simulink model "DockingSimulationModel"  (R2024b)
settings: Solver=VariableStepAuto  StartTime=0.0  StopTime=10.0  RelTol=1e-3

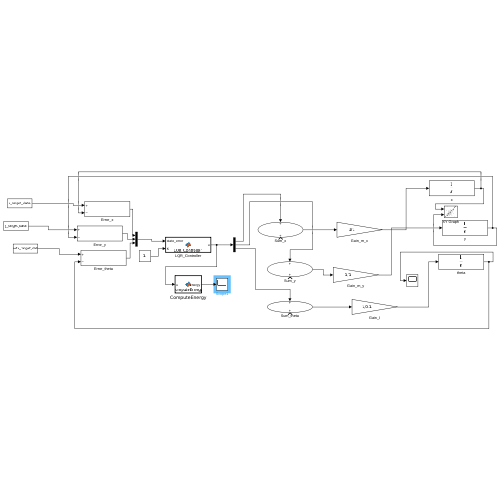
[thumbnail: Simulink's stored preview of the top-level diagram]
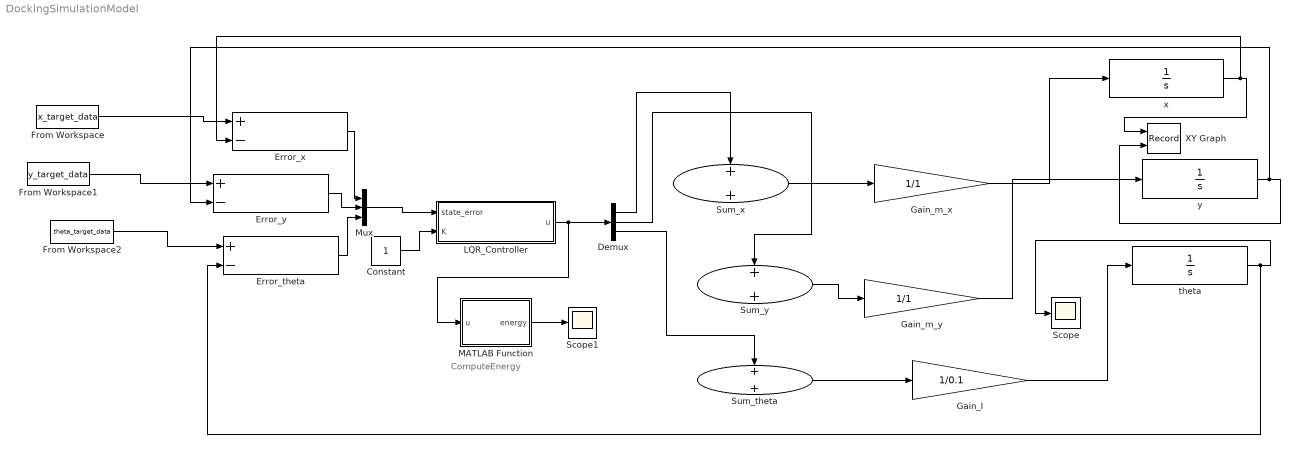
== system DockingSimulationModel ==
  note: ComputeEnergy
  Constant : Constant
  Demux : Demux  Outputs=3
  Error_theta : Sum  Inputs=+-
  Error_x : Sum  Inputs=+-
  Error_y : Sum  Inputs=+-
  From Workspace : FromWorkspace  VariableName=x_target_data
  From Workspace1 : FromWorkspace  VariableName=y_target_data
  From Workspace2 : FromWorkspace  VariableName=theta_target_data
  Gain_I : Gain  Gain=1/0.1
  Gain_m_x : Gain  Gain=1/1
  Gain_m_y : Gain  Gain=1/1
  LQR_Controller : MATLAB Function  TreatAsAtomicUnit=on
  MATLAB Function : MATLAB Function  TreatAsAtomicUnit=on
  Mux : Mux  Inputs=3
  Scope : Scope
  Scope1 : Scope
  Sum_theta : Sum
  Sum_x : Sum
  Sum_y : Sum
  XY Graph : Record  FileSettingsInternal="{\"entries\":[{\"content\":{\"excelSettings\":{\"content\":{},\"type\":\"Streamout.ExcelSettings\"}},\"type\":\"Streamout.FileSettingStorage\",\"uuid\":\"\"}],\"packageUris\":[\"http:\\/\\/schema.mathworks.com\\/mf0\\/streamout_blocks\\/R2020a\"],\"version\":\"1.0\"}"  Layout=[1 1]  SignalsInternal="{\"entries\":[{\"content\":{\"signals\":[{\"content\":{\"blockPath\":[],\"dimensions\":[1,1],\"domain\":\"\",\"lineColor\":\"#a2142f\",\"plots\":[ 1 ],\"port\":1,\"sid\":[\"\"],\"signalID\":1,\"signalName\":\"x\"},\"type\":\"RecordBlkView.Signal\",\"uuid\":\"\"},{\"content\":{\"blockPath\":[],\"dimensions\":[1,1],\"domain\":\"\",\"lineColor\":\"#139fff\",\"plots\":[ 1 ],\"port\":2,\"sid\":[\"\"],\"signalID\":2,\"signalName\":\"y\"},\"type\":\"RecordBlkView.Signal\",\"uuid\":\"\"}]},\"type\":\"RecordBlkView.InputSignals\",\"uuid\":\"\"}],\"packageUris\":[\"http:\\/\\/schema.mathworks.com\\/mf0\\/streamout_blocks\\/R2020a\"],\"version\":\"1.0\"}"  VisualizationBindings="{\"xyplotplugin\":{\"info\":[{\"series\":[{\"bindingParametersList\":[{\"parameter\":\"X-Axis\",\"signalID\":1,\"signalName\":\"x\"},{\"parameter\":\"Y-Axis\",\"signalID\":2,\"signalName\":\"y\"}],\"seriesID\":0}],\"subplotID\":1}]}}"  CompatibilityTag=XY
  theta : Integrator
  x : Integrator
  y : Integrator
  wires:
  LQR_Controller/1(u) -> MATLAB Function/1(u), Demux/1
  Demux/1 -> Sum_x/1
  Demux/2 -> Sum_y/1
  Demux/3 -> Sum_theta/1
  Error_x/1 -> Mux/1
  Error_y/1 -> Mux/2
  Error_theta/1 -> Mux/3
  Mux/1 -> LQR_Controller/1(state_error)
  x/1 -> Error_x/2, XY Graph/1
  y/1 -> Error_y/2, XY Graph/2
  theta/1 -> Error_theta/2, Scope/1
  MATLAB Function/1(energy) -> Scope1/1
  Sum_x/1 -> Gain_m_x/1
  Sum_y/1 -> Gain_m_y/1
  Sum_theta/1 -> Gain_I/1
  Gain_m_x/1 -> x/1
  Gain_m_y/1 -> y/1
  Gain_I/1 -> theta/1
  Constant/1 -> LQR_Controller/2(K)
  From Workspace/1 -> Error_x/1
  From Workspace1/1 -> Error_y/1
  From Workspace2/1 -> Error_theta/1

== matlab function DockingSimulationModel/LQR_Controller ==
  data: state_error input; u output; K input
function u = LQR_Controller(state_error, K)
    % Compute control input using precomputed LQR gain
    u = -K * state_error; % Control law
end

== matlab function DockingSimulationModel/MATLAB Function ==
  settings: updateMethod=DISCRETE
  data: u input; energy output
function energy = ComputeEnergy(u)
    persistent total_energy;
    if isempty(total_energy)
        total_energy = 0;
    end
    total_energy = total_energy + sum(u.^2);
    energy = total_energy;
end
